simulink model "pwm_esp32_udp_stable"  (R2024b)
settings: Solver=FixedStepDiscrete  StartTime=0.0  StopTime=inf  FixedStep=0.001  RelTol=1e-3
libraries: dspnetwork x2
settings Model: Creator=Anny  LastModifiedBy=Anny

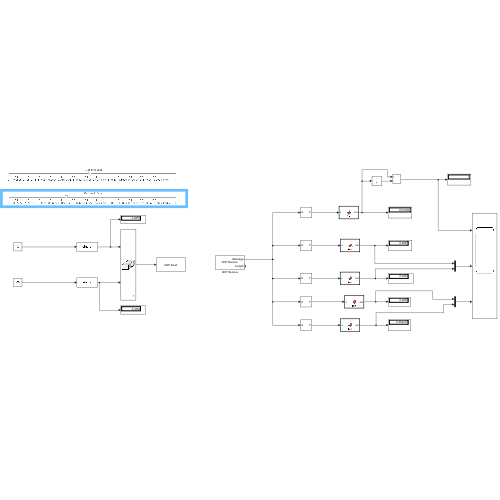
[thumbnail: Simulink's stored preview of the top-level diagram]
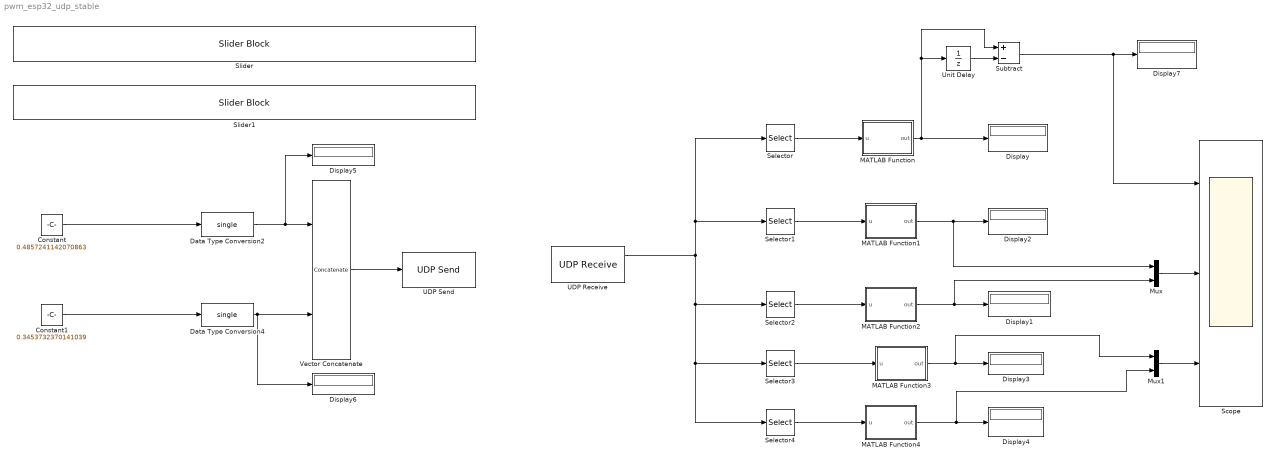
== system pwm_esp32_udp_stable ==
  Constant : Constant  Value=0.4857241142070863
  Constant1 : Constant  Value=0.3453732370141039
  Data Type Conversion2 : DataTypeConversion  OutDataTypeStr=single  SaturateOnIntegerOverflow=off  RndMeth=Floor
  Data Type Conversion4 : DataTypeConversion  OutDataTypeStr=single  SaturateOnIntegerOverflow=off  RndMeth=Floor
  Display{,1..7} (8 alike) : Display
  MATLAB Function : MATLAB Function  TreatAsAtomicUnit=on
  MATLAB Function1 : MATLAB Function  TreatAsAtomicUnit=on
  MATLAB Function2 : MATLAB Function  TreatAsAtomicUnit=on
  MATLAB Function3 : MATLAB Function  TreatAsAtomicUnit=on
  MATLAB Function4 : MATLAB Function  TreatAsAtomicUnit=on
  Mux : Mux  Inputs=2
  Mux1 : Mux  Inputs=2
  Scope : Scope  NumInputPorts=3
  Selector : Selector  InputPortWidth=20  IndexOptions=Index vector (dialog)  Indices=[1 2 3 4]  OutputSizes=1
  Selector1 : Selector  InputPortWidth=20  IndexOptions=Index vector (dialog)  Indices=[5 6 7 8]  OutputSizes=1
  Selector2 : Selector  InputPortWidth=20  IndexOptions=Index vector (dialog)  Indices=[9 10 11 12]  OutputSizes=1
  Selector3 : Selector  InputPortWidth=20  IndexOptions=Index vector (dialog)  Indices=[13 14 15 16]  OutputSizes=1
  Selector4 : Selector  InputPortWidth=20  IndexOptions=Index vector (dialog)  Indices=[17 18 19 20]  OutputSizes=1
  Slider : SliderBlock  ScaleMax=1
  Slider1 : SliderBlock  ScaleMax=1
  Subtract : Sum  Inputs=+-
  UDP Receive : dspnetwork/UDP Receive  localURL='0.0.0.0'  localPort=25001  remoteURL='0.0.0.0'  remotePort=-1  recvBufferSize=1024  dims=20  signalDatatype=uint8  isComplex=off  isVarSize=off  showBlockingTime=off  blockingTime=0  sampletime=0.01  blockPlatform=[]
      settings: LibrarySourceBlock=dspsrcs4/UDP Receive
  UDP Send : dspnetwork/UDP Send  remoteURL='172.20.10.2'  remotePort=12345  localURL='0.0.0.0'  localPortSource=Specify via dialog  localPort=25001  sendBufferSize=1024  sampletime=-1  blockPlatform=[]  separateLengthPort=0
      settings: LibrarySourceBlock=dspsnks4/UDP Send
  Unit Delay : UnitDelay  SampleTime=-1  HasFrameUpgradeWarning=on
  Vector Concatenate : Concatenate  Mode=Multidimensional array
  wires:
  Data Type Conversion4/1 -> Display6/1, Vector Concatenate/2
  Data Type Conversion2/1 -> Display5/1, Vector Concatenate/1
  Vector Concatenate/1 -> UDP Send/1
  MATLAB Function2/1(out) -> Mux/2, Display1/1
  Selector/1 -> MATLAB Function/1(u)
  Selector2/1 -> MATLAB Function2/1(u)
  Selector1/1 -> MATLAB Function1/1(u)
  Selector4/1 -> MATLAB Function4/1(u)
  MATLAB Function4/1(out) -> Mux1/2, Display4/1
  UDP Receive/1 -> Selector4/1, Selector3/1, Selector2/1, Selector1/1, Selector/1
  MATLAB Function/1(out) -> Subtract/1, Unit Delay/1, Display/1
  MATLAB Function1/1(out) -> Mux/1, Display2/1
  Selector3/1 -> MATLAB Function3/1(u)
  MATLAB Function3/1(out) -> Mux1/1, Display3/1
  Constant/1 -> Data Type Conversion2/1
  Constant1/1 -> Data Type Conversion4/1
  Unit Delay/1 -> Subtract/2
  Subtract/1 -> Display7/1, Scope/1
  Mux/1 -> Scope/2
  Mux1/1 -> Scope/3

== matlab function pwm_esp32_udp_stable/MATLAB Function ==
  data: u input uint8 size=[4 1]; out output single size=[1 1]
function out = fcn(u)
%#codegen
% u: [4x1] uint8
% out: single scalar

coder.varsize('out', [1 1], [0 0]); % 明确输出大小
out = typecast(uint8(u), 'single'); % 小端字节序转换
end

== matlab function pwm_esp32_udp_stable/MATLAB Function2 ==
  data: u input uint8 size=[4 1]; out output single size=[1 1]
function out = fcn(u)
%#codegen
% u: [4x1] uint8
% out: single scalar

coder.varsize('out', [1 1], [0 0]); % 明确输出大小
out = typecast(uint8(u), 'single'); % 小端字节序转换
end

== matlab function pwm_esp32_udp_stable/MATLAB Function3 ==
  data: u input uint8 size=[4 1]; out output single size=[1 1]
function out = fcn(u)
%#codegen
% u: [4x1] uint8
% out: single scalar

coder.varsize('out', [1 1], [0 0]); % 明确输出大小
out = typecast(uint8(u), 'single'); % 小端字节序转换
end

== matlab function pwm_esp32_udp_stable/MATLAB Function4 ==
  data: u input uint8 size=[4 1]; out output single size=[1 1]
function out = fcn(u)
%#codegen
% u: [4x1] uint8
% out: single scalar

coder.varsize('out', [1 1], [0 0]); % 明确输出大小
out = typecast(uint8(u), 'single'); % 小端字节序转换
end

== matlab function pwm_esp32_udp_stable/MATLAB Function1 ==
  data: u input uint8 size=[4 1]; out output single size=[1 1]
function out = fcn(u)
%#codegen
% u: [4x1] uint8
% out: single scalar

coder.varsize('out', [1 1], [0 0]); % 明确输出大小
out = typecast(uint8(u), 'single'); % 小端字节序转换
end
